simulink library "MIL_Test"  (Simulink 7.0)
values from neighbouring files (symbols this model uses):
  TID = min('TI' == AFT(1:2))    [PAS_callback.m]    (also in PSTID_callback.m = [block '/TID'])
undefined symbols (not defined in the file or in its folder): getdatatypespecs, slcm, StepSize
libraries: simulink x71, MIL_Test x6
(part 2 of 11)

== system MIL_Test/Test Data/Feature generation/Generate  local maximum  with given slope ==
  Clock : Clock
      settings: DisableCoverage=on  Decimation=10
  Limited Ramp Increasing : Subsystem
  Limited Ramp  Decreasing1 : Subsystem
  Logical Operator : Logic  AllPortsSameDT=off  OutDataTypeMode=boolean
  NoStartOfSignal1 : Switch  Criteria=u2 > Threshold
  RO : RelationalOperator  Operator=<  LogicOutDataTypeMode=boolean
  Sum : Sum  Inputs=|++  OutDataType=sfix(16)  OutScaling=2^0
  XO : Constant  DisableCoverage=on  Value=X0  OutDataType=sfix(16)  OutScaling=2^0
  XO1 : Constant  DisableCoverage=on  Value=X0  OutDataType=sfix(16)  OutScaling=2^0
  startTimeOfMax : Constant  DisableCoverage=on  Value=maxt  OutDataType=sfix(16)  OutScaling=2^0
  stopped : RelationalOperator  Operator=>  LogicOutDataTypeMode=boolean
  Maximum : Outport  OutDataType=sfix(16)  OutScaling=2^0
  wires:
  Logical Operator/1 -> NoStartOfSignal1/2
  stopped/1 -> Logical Operator/2
  RO/1 -> Logical Operator/1
  XO1/1 -> RO/2
  startTimeOfMax/1 -> stopped/2
  Clock/1 -> stopped/1
  Limited Ramp Increasing/2(MaxValue2) -> Limited Ramp  Decreasing1/1(InitialValue)
  Limited Ramp Increasing/1(Out2) -> Sum/1
  NoStartOfSignal1/1 -> Maximum/1
  XO/1 -> NoStartOfSignal1/1
  Sum/1 -> NoStartOfSignal1/3
  Limited Ramp  Decreasing1/1(Out1) -> RO/1, Sum/2

== system MIL_Test/Test Data/Feature generation/Generate  local maximum = maxvalue  @ given time ==
  Repeating Sequence : simulink/Sources/Repeating Sequence  SystemSampleTime=-1  rep_seq_t=[0 maxt maxt+1]  rep_seq_y=[X0 maxv X0]
  Maximum : Outport  OutDataType=sfix(16)  OutScaling=2^0
  wires:
  Repeating Sequence/1 -> Maximum/1

== system MIL_Test/Test Data/Feature generation/Generate any step response  characteristics ==
  Plant : TransferFcn  Numerator=[10]  Denominator=[1 1 10]
  Scope : Scope  NumInputPorts=5
      settings: YMin=-5~-5~-5~-5~-5  YMax=5~5~5~5~5  MaxDataPoints=1115000
  Step1 : Step  Time=2  SampleTime=0
  Sum : Sum  Inputs=|+-  OutDataType=sfix(16)  OutScaling=2^0
  Step response : Outport  OutDataType=sfix(16)  OutScaling=2^0
  wires:
  Sum/1 -> Plant/1
  Step1/1 -> Sum/1  "Step"
  Plant/1 -> Step response/1, Sum/2, Scope/1  "Step response"

== system MIL_Test/Test Data/Feature generation/Generate complete step ==
  InOut Bus : Inport  OutDataType=sfix(16)  OutScaling=2^0
  Bus Selector : BusSelector  OutputSignals=signal2.T
  Clock1 : Clock
      settings: Decimation=10
  Data Store : DataStoreMemory  StartFcn=triggerTime=triggerTime +50;  DataStoreName=triggerTime  OutDataType=sfix(16)  OutScaling=2^0
  Generate step : Step  InitFcn=triggerTime=0;  StartFcn=triggerTime=triggerTime+50;  Time=150  Before=100  After=40  SampleTime=0
  Generate step1 : Step  Time=100  Before=80  After=100  SampleTime=0
  Hold Time : Subsystem  TreatAsAtomicUnit=on
  Hold Value : Subsystem  TreatAsAtomicUnit=on
  Memory : Memory
  Relational Operator : RelationalOperator  Operator===  LogicOutDataTypeMode=boolean
  Switch : Switch  Criteria=u2 > Threshold
  triggered : Constant  OutDataType=sfix(16)  OutScaling=2^0
  v_Des : Outport  OutDataType=sfix(16)  OutScaling=2^0
  wires:
  Bus Selector/1 -> Memory/1  "<T>"
  Memory/1 -> Relational Operator/1
  Clock1/1 -> Hold Time/1(Clock)
  Hold Value/1(v_Des) -> Switch/2
  Switch/1 -> v_Des/1
  Generate step1/1 -> Switch/3
  Generate step/1 -> Switch/1
  Relational Operator/1 -> Hold Time/Enable, Hold Value/Enable, Hold Value/1(In1)
  triggered/1 -> Relational Operator/2
  InOut Bus/1 -> Bus Selector/1

== system MIL_Test/Test Data/Feature generation/Generate linear relation ==
  Clock : Clock
      settings: DisableCoverage=on  Decimation=10
  Product : Product  DisableCoverage=on  OutDataType=sfix(16)  OutScaling=2^0  SaturateOnIntegerOverflow=on  InputSameDT=on
  Step : Step  DisableCoverage=on  Time=0  After=c  SampleTime=0
  Out1 : Outport  OutDataType=sfix(16)  OutScaling=2^0
  wires:
  Clock/1 -> Product/2
  Product/1 -> Out1/1
  Step/1 -> Product/1

== system MIL_Test/Test Data/Feature generation/Generate min to date ==
  Sine Wave : Sin  SampleTime=0
  Step1 : Step  Time=2  SampleTime=0
  Step2 : Step  Time=5  Before=up  After=low  SampleTime=0
  Sum : Sum  Inputs=|+++  OutDataType=sfix(16)  OutScaling=2^0
  Min to date : Outport  OutDataType=sfix(16)  OutScaling=2^0
  wires:
  Step1/1 -> Sum/1  "Step"
  Sum/1 -> Min to date/1
  Step2/1 -> Sum/2
  Sine Wave/1 -> Sum/3

== system MIL_Test/Test Data/Feature generation/Generate peaks ==
  Repeating Sequence : simulink/Sources/Repeating Sequence  SystemSampleTime=-1  rep_seq_t=[0 1/freq]  rep_seq_y=[Sens -Sens]
  Peak : Outport  OutDataType=sfix(16)  OutScaling=2^0
  wires:
  Repeating Sequence/1 -> Peak/1

== system MIL_Test/Test Data/Feature generation/Generate signal  crossing a given value  @ given time ==
  Step : Step  Time=time  Before=up-low+1  After=val  SampleTime=0
  Feature : Outport  OutDataType=sfix(16)  OutScaling=2^0
  wires:
  Step/1 -> Feature/1

== system MIL_Test/Test Data/Feature generation/Generate signal which  starts to be constant @ time ==
  Clock1 : Clock
      settings: Decimation=10
  Constant : Constant  Value=const  OutDataType=sfix(16)  OutScaling=2^0
  Relational Operator : RelationalOperator  LogicOutDataTypeMode=boolean
  Sine Wave : Sin  SampleTime=0
  Switch1 : Switch  Criteria=u2 > Threshold
  start time : Constant  Value=ST  OutDataType=sfix(16)  OutScaling=2^0
  Feature : Outport  OutDataType=sfix(16)  OutScaling=2^0
  wires:
  Clock1/1 -> Relational Operator/1
  start time/1 -> Relational Operator/2
  Relational Operator/1 -> Switch1/2
  Constant/1 -> Switch1/1
  Sine Wave/1 -> Switch1/3
  Switch1/1 -> Feature/1

== system MIL_Test/Test Data/Feature generation/Generate timed constant ==
  Repeating Sequence : Subsystem  mask(Repeating table){rep_seq_t=[0 T], rep_seq_y=[X0 X0]}
      mask prompts: rep_seq_t "Time values:"; rep_seq_y "Output values:"
      mask help: Output a repeating sequence of numbers specified in a table of time-value pairs. Values of time should be monotonically increasing.
      mask init:
      | if (length(rep_seq_t) ~= length(rep_seq_y)),
      |   error('Length of time vector and output vector must be the same.')
      | end
      | dbl_rep_seq_t = double(rep_seq_t);
      | dbl_rep_seq_y = double(rep_seq_y);
      | period = max(dbl_rep_seq_t) - min(dbl_rep_seq_t);
      | s = round(length(dbl_rep_seq_t)/50);
      | if s > 0
      |   pts = [1:s:length(dbl_rep_seq_t)];
      |   L   = length(pts);
      | else
      |   L   = length(dbl_rep_seq_t);
      |   pts = [1:L];
      | end
      | 
      | disp_seq_t = reshape(dbl_rep_seq_t(pts),L,1);
      | disp_seq_y = reshape(dbl_rep_seq_y(pts),L,1);
      | disp_period = max(disp_seq_t) - min(disp_seq_t);
      | 
      | disp_seq_t  = repmat(disp_seq_t,1,3) + (ones(L,1)*(disp_period*[0,1,2]));
      | disp_seq_t = [ disp_seq_t(:); disp_seq_t(end) ];
      | disp_seq_y = repmat(disp_seq_y,1,3);
      | disp_seq_y = [ disp_seq_y(:); disp_seq_y(1) ];
      mask Help: Repeats cycle given in table. Time values should be monotonically increasing.
      mask Display: plot( disp_seq_t, disp_seq_y )
  Out1 : Outport  OutDataType=sfix(16)  OutScaling=2^0
  wires:
  Repeating Sequence/1(Out1) -> Out1/1

== system MIL_Test/Test Data/Feature generation/Generate timed limited decrease ==
  Clock : Clock
      settings: Decimation=10
  Constant : Constant  Value=start  OutDataType=sfix(16)  OutScaling=2^0
  Constant1 : Constant  Value=X0  OutDataType=sfix(16)  OutScaling=2^0
  Constant2 : Constant  Value=XF  OutDataType=sfix(16)  OutScaling=2^0
  Output : Sum  Inputs=|++  OutDataType=sfix(16)  OutScaling=2^0  SaturateOnIntegerOverflow=on  InputSameDT=on
  Product : Product  OutDataType=sfix(16)  OutScaling=2^0  SaturateOnIntegerOverflow=on  InputSameDT=on
  Step : Step  Time=start  After=(XF-X0)/T  SampleTime=0
  Subsystem : Subsystem
  Sum : Sum  Inputs=|+-  OutDataType=sfix(16)  OutScaling=2^0  SaturateOnIntegerOverflow=on  InputSameDT=on
  Out1 : Outport  OutDataType=sfix(16)  OutScaling=2^0
  wires:
  Constant2/1 -> Subsystem/1(In1)
  Step/1 -> Product/1
  Product/1 -> Output/1
  Constant1/1 -> Output/2, Subsystem/3(In3)
  Output/1 -> Subsystem/2(In2)
  Sum/1 -> Product/2
  Constant/1 -> Sum/2
  Clock/1 -> Sum/1
  Subsystem/1(Out1) -> Out1/1

== system MIL_Test/Test Data/Feature generation/Generate timed limited increase ==
  Clock : Clock
      settings: Decimation=10
  Constant : Constant  Value=start  OutDataType=sfix(16)  OutScaling=2^0
  Constant1 : Constant  Value=X0  OutDataType=sfix(16)  OutScaling=2^0
  Constant2 : Constant  Value=XF  OutDataType=sfix(16)  OutScaling=2^0
  Output : Sum  Inputs=|++  OutDataType=sfix(16)  OutScaling=2^0  SaturateOnIntegerOverflow=on  InputSameDT=on
  Product : Product  OutDataType=sfix(16)  OutScaling=2^0  SaturateOnIntegerOverflow=on  InputSameDT=on
  Step : Step  Time=start  After=(XF-X0)/T  SampleTime=0
  Subsystem : Subsystem
  Sum : Sum  Inputs=|+-  OutDataType=sfix(16)  OutScaling=2^0  SaturateOnIntegerOverflow=on  InputSameDT=on
  Out1 : Outport  OutDataType=sfix(16)  OutScaling=2^0
  wires:
  Step/1 -> Product/1
  Product/1 -> Output/1
  Constant1/1 -> Output/2, Subsystem/3(In3)
  Sum/1 -> Product/2
  Constant/1 -> Sum/2
  Clock/1 -> Sum/1
  Constant2/1 -> Subsystem/1(In1)
  Output/1 -> Subsystem/2(In2)  "U(k)"
  Subsystem/1(Out1) -> Out1/1

== system MIL_Test/Test Data/Signal comparison/Bound Precond ==
  Signal : Inport  OutDataType=sfix(16)  OutScaling=2^0
  Reference : Inport  Port=2  OutDataType=sfix(16)  OutScaling=2^0
  RelOp : RelationalOperator  LogicOutDataTypeMode=Specify via dialog
  Activate : Outport  OutDataType=sfix(16)  OutScaling=2^0
  wires:
  Reference/1 -> RelOp/2
  RelOp/1 -> Activate/1
  Signal/1 -> RelOp/1

== system MIL_Test/Test Data/Signal comparison/Range - Gap Absolute tolerance Precond ==
  Signal : Inport  OutDataType=sfix(16)  OutScaling=2^0
  Reference : Inport  Port=2  OutDataType=sfix(16)  OutScaling=2^0
  Abs : Abs
  Abs1 : Abs
  Absolute Tolerance : Constant  Value=AbsoluteTolerance  OutDataType=sfix(16)  OutScaling=2^0
  Add : Sum  Inputs=+-  OutDataType=sfix(16)  OutScaling=2^-10
  Relational Operator : RelationalOperator  Operator===  LogicOutDataTypeMode=boolean
  Activate : Outport  OutDataType=sfix(16)  OutScaling=2^0
  wires:
  Abs1/1 -> Relational Operator/2
  Absolute Tolerance/1 -> Abs1/1
  Reference/1 -> Add/2
  Signal/1 -> Add/1
  Add/1 -> Abs/1
  Abs/1 -> Relational Operator/1
  Relational Operator/1 -> Activate/1

== system MIL_Test/Test Data/Signal comparison/Range - Gap Relative tolerance Precond ==
  Signal : Inport  OutDataType=sfix(16)  OutScaling=2^0
  Reference : Inport  Port=2  OutDataType=sfix(16)  OutScaling=2^0
  Abs : Abs
  Abs1 : Abs
  Add : Sum  Inputs=+-  OutDataType=sfix(16)  OutScaling=2^-10
  Divide1 : Product  Inputs=**/  OutDataType=sfix(16)  OutScaling=2^-10
  Max : Constant  Value=100  OutDataType=sfix(16)  OutScaling=2^0
  Relational Operator : RelationalOperator  Operator=<=  LogicOutDataTypeMode=boolean
  Relative Tolerance : Constant  OutDataType=sfix(16)  OutScaling=2^0
  Activate : Outport  OutDataType=sfix(16)  OutScaling=2^0
  wires:
  Abs/1 -> Relational Operator/1
  Add/1 -> Abs/1
  Signal/1 -> Add/1
  Reference/1 -> Add/2, Abs1/1
  Divide1/1 -> Relational Operator/2
  Max/1 -> Divide1/3
  Relative Tolerance/1 -> Divide1/2
  Relational Operator/1 -> Activate/1
  Abs1/1 -> Divide1/1

== system MIL_Test/Test Data/Signal comparison/Range - Gap Tolerance range Precond ==
  Signal : Inport  OutDataType=sfix(16)  OutScaling=2^0
  Lower bound : Inport  Port=2  OutDataType=sfix(16)  OutScaling=2^0
  Upper bound : Inport  Port=3  OutDataType=sfix(16)  OutScaling=2^0
  Logical Operator : Logic  AllPortsSameDT=off  OutDataTypeMode=Specify via dialog
  Relational Operator : RelationalOperator  LogicOutDataTypeMode=boolean
  Relational Operator1 : RelationalOperator  LogicOutDataTypeMode=boolean
  Activate : Outport  OutDataType=sfix(16)  OutScaling=2^0
  wires:
  Upper bound/1 -> Relational Operator1/1
  Relational Operator/1 -> Logical Operator/2
  Relational Operator1/1 -> Logical Operator/1
  Signal/1 -> Relational Operator/1, Relational Operator1/2
  Logical Operator/1 -> Activate/1
  Lower bound/1 -> Relational Operator/2

== system MIL_Test/Test Data/Test Data Architecture/<Test data generator> ==
  Test Ctrl Influence : Inport  OutDataType=sfix(16)  OutScaling=2^0
  Out Bus : Inport  Port=2  OutDataType=sfix(16)  OutScaling=2^0
  <Requirement name> : Subsystem
  switch <signal1> : MultiPortSwitch  Inputs=1  zeroidx=on
  <signal1> : Outport  OutDataType=sfix(16)  OutScaling=2^0
  wires:
  Test Ctrl Influence/1 -> switch <signal1>/1
  Out Bus/1 -> <Requirement name>/1(Out Bus)
  switch <signal1>/1 -> <signal1>/1
  <Requirement name>/1(<signal1>) -> switch <signal1>/2

== system MIL_Test/Test Quality/VFs Activation  Coverage/Max to date ==
  Signal : Inport  OutDataType=sfix(16)  OutScaling=2^0
  Clock : Clock
      settings: Decimation=10
  Memory : Memory  Orientation=left
  MinMax : MinMax  Function=max  Inputs=2  OutDataType=sfix(16)  OutScaling=2^0
  Switch : Switch  Criteria=u2 > Threshold
  Max : Outport  OutDataType=sfix(16)  OutScaling=2^0
  wires:
  Memory/1 -> Switch/1
  Clock/1 -> Switch/2
  Switch/1 -> MinMax/1
  Signal/1 -> Switch/3, MinMax/2
  MinMax/1 -> Memory/1, Max/1

== system MIL_Test/Test Quality/VFs Activation  Coverage/Max to date1 ==
  Signal : Inport  OutDataType=sfix(16)  OutScaling=2^0
  Clock : Clock
      settings: Decimation=10
  Memory : Memory  Orientation=left
  MinMax : MinMax  Function=max  Inputs=2  OutDataType=sfix(16)  OutScaling=2^0
  Switch : Switch  Criteria=u2 > Threshold
  Max : Outport  OutDataType=sfix(16)  OutScaling=2^0
  wires:
  Memory/1 -> Switch/1
  Clock/1 -> Switch/2
  Switch/1 -> MinMax/1
  Signal/1 -> Switch/3, MinMax/2
  MinMax/1 -> Memory/1, Max/1

== system MIL_Test/Validation Function/Feature extraction/Complete step detection ==
  Step : Inport  OutDataType=sfix(16)  OutScaling=2^0
  Step response : Inport  Port=2  OutDataType=sfix(16)  OutScaling=2^0
  Step detection : Subsystem  mask{MT=10, RT=0.001}
      mask prompts: MT "Minimal time for signals to be constant before a step"; RT "Relative tolerance for constant detection in %"
      mask CallbackString:
      | if (str2double(get_param(gcb,'MT')) < 0)
      |     error(['Minimal time specified (' get_param(gcb,'MT') ') negative. Please give a non-negative value.']);
      | else
      |     set_param([gcb '/Active if signals constant for some specified time/Min Time'],'Value',get_param(gcb,'MT'));
      | end|if or( (str2double(get_param(gcb,'RT')) < 0), (str2double(get_param(gcb,'RT')) > 100))
      |     error(['Relative tolerance value (' get_param(gcb,'RT') ') out of range. Please give a value between 0 and 100.']);
      | else
      |     set_param([gcb '/Active if signals constant for some specified time/Time since signal constant/Detect constant/Relative tolerance/Relative Tolerance'],'Value',get_param(gcb,'RT'));
      |     set_param([gcb '/Active if signals constant for some specified time/Time since signal constant/Detect constant'],'RT',get_param(gcb,'RT'));
      |     set_param([gcb '/Active if signals constant for some specified time/Time since signal constant'],'RT',get_param(gcb,'RT'));
      |     set_param([gcb '/Active if signals constant for some specified time/Time since signal constant1/Detect constant/Relative tolerance/Relative Tolerance'],'Value',get_param(gcb,'RT'));
      |     set_param([gcb '/Active if signals constant for some specified time/Time since signal constant1/Detect constant'],'RT',get_param(gcb,'RT'));
      |     set_param([gcb '/Active if signals constant for some specified time/Time since signal constant1'],'RT',get_param(gcb,'RT'));
      | end
  Step detection reset : Subsystem  mask{MT=10, RT=0.0001, MSS=10}
      mask prompts: MT "Minimal time for signals to be constant before a step"; RT "Relative tolerance for constant detection in %"; MSS "Minimal step size for step detection"
      mask CallbackString:
      | if (str2double(get_param(gcb,'MT')) < 0)
      |     error(['Minimal time specified (' get_param(gcb,'MT') ') negative. Please give a non-negative value.']);
      | else
      |     set_param([gcb '/Active if signals constant for some specified time/Min Time'],'Value',get_param(gcb,'MT'));
      | end|if or( (str2double(get_param(gcb,'RT')) < 0), (str2double(get_param(gcb,'RT')) > 100))
      |     error(['Relative tolerance value (' get_param(gcb,'RT') ') out of range. Please give a value between 0 and 100.']);
      | else
      |     set_param([gcb '/Active if signals constant for some specified time/Time since signal constant/Detect constant/Relative tolerance/Relative Tolerance'],'Value',get_param(gcb,'RT'));
      |     set_param([gcb '/Active if signals constant for some specified time/Time since signal constant/Detect constant'],'RT',get_param(gcb,'RT'));
      |     set_param([gcb '/Active if signals constant for some specified time/Time since signal constant'],'RT',get_param(gcb,'RT'));
      |     set_param([gcb '/Active if signals constant for some specified time/Time since signal constant1/Detect constant/Relative tolerance/Relative Tolerance'],'Value',get_param(gcb,'RT'));
      |     set_param([gcb '/Active if signals constant for some specified time/Time since signal constant1/Detect constant'],'RT',get_param(gcb,'RT'));
      |     set_param([gcb '/Active if signals constant for some specified time/Time since signal constant1'],'RT',get_param(gcb,'RT'));
      | end|if (str2double(get_param(gcb,'MSS')) < 0)
      |     error(['Minimal step size specified (' get_param(gcb,'MSS') ') negative. Please give a non-negative value.']);
      | else
      |     set_param([gcb '/Step detection/Min step size'],'Value',get_param(gcb,'MSS'));
      |     set_param([gcb '/Step detection'],'StepSize',get_param(gcb,'MSS'));
      | 
      | end
  R : Outport  OutDataType=sfix(16)  OutScaling=2^0
  T : Outport  Port=2  OutDataType=sfix(16)  OutScaling=2^0
  Complete step : Outport  Port=3  OutDataType=sfix(16)  OutScaling=2^0
  wires:
  Step detection/1(End of complete step) -> T/1, Complete step/1
  Step detection reset/1(R) -> R/1, Step detection/1(R)
  Step response/1 -> Step detection reset/2(Step response), Step detection/3(Step response)
  Step/1 -> Step detection reset/1(Step), Step detection/2(Step)

== system MIL_Test/Validation Function/Feature extraction/Detect constant ==
  Signal : Inport  OutDataType=sfix(16)  OutScaling=2^0
  Clock : Clock
      settings: Decimation=10
  Constant1 : Constant  Value=0  OutDataTypeMode=boolean  OutDataType=sfix(16)  OutScaling=2^0
  Memory : Memory
  Relative tolerance : Subsystem
  Switch : Switch  Criteria=u2 > Threshold
  Constant : Outport  OutDataType=sfix(16)  OutScaling=2^0
  wires:
  Switch/1 -> Constant/1
  Relative tolerance/1(sig == ref) -> Switch/1
  Clock/1 -> Switch/2
  Constant1/1 -> Switch/3
  Memory/1 -> Relative tolerance/2(ref)
  Signal/1 -> Relative tolerance/1(sig), Memory/1

== system MIL_Test/Validation Function/Feature extraction/Detect decrease ==
  Signal : Inport  OutDataType=sfix(16)  OutScaling=2^0
  Clock : Clock
      settings: Decimation=10
  Memory : Memory
  Relational Operator : RelationalOperator  Operator=<  LogicOutDataTypeMode=Specify via dialog
  Switch : Switch  Criteria=u2 > Threshold
  Decrease : Outport  OutDataType=sfix(16)  OutScaling=2^0
  wires:
  Signal/1 -> Relational Operator/1, Memory/1, Switch/3
  Relational Operator/1 -> Decrease/1
  Clock/1 -> Switch/2
  Memory/1 -> Switch/1
  Switch/1 -> Relational Operator/2

== system MIL_Test/Validation Function/Feature extraction/Detect increase ==
  Signal : Inport  OutDataType=sfix(16)  OutScaling=2^0
  Clock : Clock
      settings: Decimation=10
  Memory : Memory
  Relational Operator : RelationalOperator  Operator=>  LogicOutDataTypeMode=Specify via dialog
  Switch : Switch  Criteria=u2 > Threshold
  Increase : Outport  OutDataType=sfix(16)  OutScaling=2^0
  wires:
  Switch/1 -> Relational Operator/2
  Memory/1 -> Switch/1
  Clock/1 -> Switch/2
  Relational Operator/1 -> Increase/1
  Signal/1 -> Switch/3, Memory/1, Relational Operator/1

== system MIL_Test/Validation Function/Feature extraction/Linear relation ==
  y : Inport  OutDataType=sfix(16)  OutScaling=2^0
  u : Inport  Port=2  OutDataType=sfix(16)  OutScaling=2^0
  Product : Product  OutDataType=sfix(16)  OutScaling=2^0  RndMeth=Zero
  Relative tolerance : Subsystem
  c : Constant  Value=5  OutDataType=sfix(16)  OutScaling=2^0
  y == c u : Outport  OutDataType=sfix(16)  OutScaling=2^0
  wires:
  Relative tolerance/1(sig == ref) -> y == c u/1
  c/1 -> Product/2
  u/1 -> Product/1
  Product/1 -> Relative tolerance/2(ref)
  y/1 -> Relative tolerance/1(sig)

== system MIL_Test/Validation Function/Feature extraction/Local maximum ==
  Signal : Inport  OutDataType=sfix(16)  OutScaling=2^0
  Clock : Clock
      settings: Decimation=10
  Clock1 : Clock
      settings: Decimation=10
  Logical Operator : Logic  AllPortsSameDT=off  OutDataTypeMode=boolean
  Memory : Memory
  Memory1 : Memory
  Relational Operator : RelationalOperator  Operator=<  LogicOutDataTypeMode=boolean
  Relational Operator1 : RelationalOperator  Operator=>  LogicOutDataTypeMode=boolean
  Switch : Switch  Criteria=u2 > Threshold
  Switch1 : Switch  Criteria=u2 > Threshold
  Maximum : Outport  OutDataType=sfix(16)  OutScaling=2^0
  wires:
  Switch1/1 -> Relational Operator1/2
  Memory1/1 -> Switch1/1
  Clock1/1 -> Switch1/2
  Switch/1 -> Relational Operator1/1, Switch1/3, Memory1/1, Relational Operator/2
  Memory/1 -> Switch/1
  Clock/1 -> Switch/2
  Relational Operator/1 -> Logical Operator/1
  Relational Operator1/1 -> Logical Operator/2
  Logical Operator/1 -> Maximum/1
  Signal/1 -> Switch/3, Memory/1, Relational Operator/1

== system MIL_Test/Validation Function/Feature extraction/Min to date ==
  Signal : Inport  OutDataType=sfix(16)  OutScaling=2^0
  Clock : Clock
      settings: Decimation=10
  Memory : Memory  Orientation=left
  MinMax : MinMax  Inputs=2  OutDataType=sfix(16)  OutScaling=2^0
  Switch : Switch  Criteria=u2 > Threshold
  Min : Outport  OutDataType=sfix(16)  OutScaling=2^0
  wires:
  Memory/1 -> Switch/1
  Clock/1 -> Switch/2
  Switch/1 -> MinMax/1
  Signal/1 -> Switch/3, MinMax/2
  MinMax/1 -> Memory/1, Min/1

== system MIL_Test/Validation Function/Feature extraction/Moving average ==
  Signal : Inport  OutDataType=sfix(16)  OutScaling=2^0
  Add : Sum  OutDataType=sfix(16)  OutScaling=2^-10
  Clock : Clock
      settings: Decimation=10
  Constant : Constant  Value=2  OutDataType=sfix(16)  OutScaling=2^0
  Divide : Product  Inputs=*/  OutDataType=sfix(16)  OutScaling=2^-10
  Memory : Memory
  Switch : Switch  Criteria=u2 > Threshold
  MA : Outport  OutDataType=sfix(16)  OutScaling=2^0
  wires:
  Switch/1 -> Add/2
  Memory/1 -> Switch/1
  Clock/1 -> Switch/2
  Signal/1 -> Add/1, Switch/3, Memory/1
  Add/1 -> Divide/1
  Constant/1 -> Divide/2
  Divide/1 -> MA/1

== system MIL_Test/Validation Function/Feature extraction/Peak detection ==
  Signal : Inport  OutDataType=sfix(16)  OutScaling=2^0
  Abs : Abs
  Abs1 : Abs
  Add : Sum  Inputs=+-  OutDataType=sfix(16)  OutScaling=2^-10
  Add1 : Sum  Inputs=+-  OutDataType=sfix(16)  OutScaling=2^-10
  Clock : Clock
      settings: Decimation=10
  Clock1 : Clock
      settings: Decimation=10
  Compare To Zero : simulink/Logic and Bit Operations/Compare To Zero  SystemSampleTime=-1  relop=<=  LogicOutDataTypeMode=boolean  ZeroCross=off
  Logical Operator : Logic  Inputs=3  AllPortsSameDT=off  OutDataTypeMode=boolean
  Memory : Memory
  Memory1 : Memory
  Product : Product  OutDataType=sfix(16)  OutScaling=2^0  RndMeth=Zero
  Relational Operator : RelationalOperator  Operator=<=  LogicOutDataTypeMode=boolean
  Relational Operator1 : RelationalOperator  LogicOutDataTypeMode=boolean
  Sensibility1 : Constant  Value=0.198  OutDataType=sfix(16)  OutScaling=2^0
  Sensibility2 : Constant  Value=0.198  OutDataType=sfix(16)  OutScaling=2^0
  Switch : Switch  Criteria=u2 > Threshold
  Switch1 : Switch  Criteria=u2 > Threshold
  Peak : Outport  OutDataType=sfix(16)  OutScaling=2^0
  wires:
  Sensibility2/1 -> Relational Operator1/2
  Abs1/1 -> Relational Operator1/1
  Sensibility1/1 -> Relational Operator/1
  Abs/1 -> Relational Operator/2
  Product/1 -> Compare To Zero/1
  Compare To Zero/1 -> Logical Operator/2
  Relational Operator1/1 -> Logical Operator/3
  Relational Operator/1 -> Logical Operator/1
  Add1/1 -> Product/2, Abs1/1
  Signal/1 -> Memory/1, Switch/3, Add/1
  Logical Operator/1 -> Peak/1
  Clock/1 -> Switch/2
  Memory/1 -> Switch/1
  Switch/1 -> Add1/1, Add/2, Memory1/1, Switch1/3
  Clock1/1 -> Switch1/2
  Memory1/1 -> Switch1/1
  Switch1/1 -> Add1/2
  Add/1 -> Product/1, Abs/1

== system MIL_Test/Validation Function/Feature extraction/Signal value @ maximum ==
  Signal : Inport  OutDataType=sfix(16)  OutScaling=2^0
  Local maximum : Subsystem  TreatAsAtomicUnit=on
  Trigger : Outport  OutDataType=sfix(16)  OutScaling=2^0
  Feature : Outport  Port=2  OutDataType=sfix(16)  OutScaling=2^0
  wires:
  Local maximum/1(Maximum) -> Trigger/1
  Signal/1 -> Local maximum/1(Signal), Feature/1

== system MIL_Test/Validation Function/Feature extraction/Step detection ==
  Signal : Inport  OutDataType=sfix(16)  OutScaling=2^0
  Abs : Abs
  Add : Sum  Inputs=+-  OutDataType=sfix(16)  OutScaling=2^-10
  Clock : Clock
      settings: Decimation=10
  Memory : Memory
  Min step size : Constant  OutDataType=sfix(16)  OutScaling=2^0
  Relational Operator : RelationalOperator  LogicOutDataTypeMode=boolean
  Switch : Switch  Criteria=u2 > Threshold
  Step : Outport  OutDataType=sfix(16)  OutScaling=2^0
  wires:
  Switch/1 -> Add/2
  Memory/1 -> Switch/1
  Clock/1 -> Switch/2
  Signal/1 -> Add/1, Switch/3, Memory/1
  Abs/1 -> Relational Operator/1
  Min step size/1 -> Relational Operator/2
  Relational Operator/1 -> Step/1
  Add/1 -> Abs/1

== system MIL_Test/Validation Function/Feature extraction/Step response characteristics ==
  Step : Inport  OutDataType=sfix(16)  OutScaling=2^0
  Step response : Inport  Port=2  OutDataType=sfix(16)  OutScaling=2^0
  Step response characteristics extraction : Subsystem  mask(Step response feature extraction){gain=0.8333, lowerLim=10, upperLim=90, MOma=ones(1,10), RelTol=0.1, MinTime=1, Range=5, sseW=ones(1,10)}
      mask prompts: gain "System's static gain"; lowerLim "Rise time interval lower limit (in set point %)"; upperLim "Rise time interval upper limit (in set point %)"; MOma "Maximum overshoot moving average weights"; RelTol "Maximum overshoot - Detect constant if no overshoot - Relative Tolerance"; MinTime "Maximum overshoot - Detect constant if no overshoot - Minimum constant time"; Range "Settling time range (in set point %)"; sseW "Steady state error - moving average weights"
      mask help: Extracts four step response feature characteristics. Extraction parameters are shown below.
      mask CallbackString:
      | set_param([gcb '/Static Gain'],'Value',get_param(gcb,'gain'));|set_param([gcb '/Extract rise time/lowerLim'],'Value',get_param(gcb,'lowerLim'));|set_param([gcb '/Extract rise time/upperLim'],'Value',get_param(gcb,'upperLim'));|set_param([gcb '/Extract maximum overshoot/Step response moving average and initial conditions before step/Weighted Moving Average'],'mgainval',get_param(gcb,'MOma'));
      | set_param([gcb '/Extract maximum overshoot/Step response moving average and initial conditions before step/Weighted Moving Average1'],'mgainval',get_param(gcb,'MOma'));|set_param([gcb '/Extract maximum overshoot/Active if signals constant for some specified time/Time since signal constant'],'RT',get_param(gcb,'RelTol'));
      | set_param([gcb '/Extract maximum overshoot/Active if signals constant for some specified time/Time since signal constant1'],'RT',get_param(gcb,'RelTol'));|set_param([gcb '/Extract maximum overshoot/Active if signals constant for some specified time/Min Time'],'Value',get_param(gcb,'MinTime'));|set_param([gcb '/Extract settling time/Set point percent'],'Value',get_param(gcb,'Range'));|set_param([gcb '/Extract steady state error/Weighted Moving Average'],'mgainval',get_param(gcb,'sseW'));
  Step response reset : Subsystem  mask{MT=1, RT=0.0001, MSS=1}
      mask prompts: MT "Minimal time for signals to be constant before a step"; RT "Relative tolerance for constant detection in %"; MSS "Minimal step size for step detection"
      mask CallbackString:
      | if (str2double(get_param(gcb,'MT')) < 0)
      |     error(['Minimal time specified (' get_param(gcb,'MT') ') negative. Please give a non-negative value.']);
      | else
      |     set_param([gcb '/Active if signals constant for some specified time/Min Time'],'Value',get_param(gcb,'MT'));
      | end|if or( (str2double(get_param(gcb,'RT')) < 0), (str2double(get_param(gcb,'RT')) > 100))
      |     error(['Relative tolerance value (' get_param(gcb,'RT') ') out of range. Please give a value between 0 and 100.']);
      | else
      |     set_param([gcb '/Active if signals constant for some specified time/Time since signal constant/Detect constant/Relative tolerance/Relative Tolerance'],'Value',get_param(gcb,'RT'));
      |     set_param([gcb '/Active if signals constant for some specified time/Time since signal constant/Detect constant'],'RT',get_param(gcb,'RT'));
      |     set_param([gcb '/Active if signals constant for some specified time/Time since signal constant'],'RT',get_param(gcb,'RT'));
      |     set_param([gcb '/Active if signals constant for some specified time/Time since signal constant1/Detect constant/Relative tolerance/Relative Tolerance'],'Value',get_param(gcb,'RT'));
      |     set_param([gcb '/Active if signals constant for some specified time/Time since signal constant1/Detect constant'],'RT',get_param(gcb,'RT'));
      |     set_param([gcb '/Active if signals constant for some specified time/Time since signal constant1'],'RT',get_param(gcb,'RT'));
      | end|if (str2double(get_param(gcb,'MSS')) < 0)
      |     error(['Minimal step size specified (' get_param(gcb,'MSS') ') negative. Please give a non-negative value.']);
      | else
      |     set_param([gcb '/Step detection/Min step size'],'Value',get_param(gcb,'MSS'));
      |     set_param([gcb '/Step detection'],'StepSize',get_param(gcb,'MSS'));
      | 
      | end
  Step response trigger : Subsystem  mask(Step response trigger extraction){MinTime=1, RelTol=0.5, MAXsse=0.5}
      mask prompts: MinTime "Detect constant signals - Minimum constant time"; RelTol "Detect constant signals - Relative Tolerance"; MAXsse "Maximum steady state error for triggering"
      mask help: This block extracts the trigger signals for the four step response characteristics.
      mask CallbackString:
      | set_param([gcb '/Active if signals constant for some specified time/Min Time'],'Value',get_param(gcb,'MinTime'));|set_param([gcb '/Active if signals constant for some specified time/Time since signal constant'],'RT',get_param(gcb,'RelTol'));
      | set_param([gcb '/Active if signals constant for some specified time/Time since signal constant1'],'RT',get_param(gcb,'RelTol'));|set_param([gcb '/Compare To Constant'],'const',get_param(gcb,'MAXsse'));
  R : Outport  OutDataType=sfix(16)  OutScaling=2^0
  Rise time T : Outport  Port=2  DataType=double  OutDataType=sfix(16)  OutScaling=2^0
  Overshoot T : Outport  Port=3  DataType=double  OutDataType=sfix(16)  OutScaling=2^0
  Settling time T : Outport  Port=4  DataType=double  OutDataType=sfix(16)  OutScaling=2^0
  Steady state error T : Outport  Port=5  DataType=double  OutDataType=sfix(16)  OutScaling=2^0
  Rise time : Outport  Port=6  OutDataType=sfix(16)  OutScaling=2^0
  Maximum Overshoot : Outport  Port=7  OutDataType=sfix(16)  OutScaling=2^0
  Settling time : Outport  Port=8  DataType=double  OutDataType=sfix(16)  OutScaling=2^0
  Steady state error : Outport  Port=9  DataType=double  OutDataType=sfix(16)  OutScaling=2^0
  wires:
  Step response trigger/4(Steady state error T) -> Steady state error T/1
  Step response trigger/3(Settling time T) -> Settling time T/1
  Step response trigger/2(Overshoot T) -> Overshoot T/1
  Step response trigger/1(Rise time T) -> Rise time T/1
  Step response characteristics extraction/2(Maximum overshoot) -> Maximum Overshoot/1
  Step response characteristics extraction/3(Settling time) -> Settling time/1
  Step response characteristics extraction/1(Rise time) -> Rise time/1
  Step response/1 -> Step response trigger/2(Step response), Step response characteristics extraction/3(Step response), Step response reset/2(Step response)
  Step/1 -> Step response characteristics extraction/2(Step), Step response reset/1(Step)
  Step response characteristics extraction/4(Steady state error) -> Steady state error/1, Step response trigger/1(Steady state error)
  Step response reset/1(R) -> Step response characteristics extraction/1(R), R/1

== system MIL_Test/Validation Function/Feature extraction/Time @ sig = x ==
  Signal : Inport  OutDataType=sfix(16)  OutScaling=2^0
  Clock : Clock
      settings: Decimation=10
  Relative tolerance : Subsystem
  Trigger Value : Constant  Value=5  OutDataType=sfix(16)  OutScaling=2^0
  Trigger : Outport  OutDataType=sfix(16)  OutScaling=2^0
  Feature : Outport  Port=2  OutDataType=sfix(16)  OutScaling=2^0
  wires:
  Clock/1 -> Feature/1
  Trigger Value/1 -> Relative tolerance/2(ref)
  Signal/1 -> Relative tolerance/1(sig)
  Relative tolerance/1(sig == ref) -> Trigger/1

== system MIL_Test/Validation Function/Feature extraction/Time since signal constant ==
  Signal : Inport  OutDataType=sfix(16)  OutScaling=2^0
  Clock : Clock
      settings: Decimation=10
  Detect constant : Subsystem  TreatAsAtomicUnit=on  mask(Feature extraction block){RT=1}
      mask prompts: RT "Relative tolerance in %"
      mask help: Detect if the signal value is constant (using the last two signal values) allowing for a user-defined relative deviation
      mask CallbackString:
      | if or( (str2double(get_param(gcb,'RT')) < 0), (str2double(get_param(gcb,'RT')) > 100))
      |     error(['Relative tolerance value (' get_param(gcb,'RT') ') out of range. Please give a value between 0 and 100.']);
      | else
      |     set_param([gcb '/Relative tolerance/Relative Tolerance'],'Value',get_param(gcb,'RT'));
      | end
  Logical Operator : Logic  Operator=NAND  AllPortsSameDT=off  OutDataTypeMode=boolean
  Logical Operator1 : Logic  Operator=NOT  AllPortsSameDT=off  OutDataTypeMode=boolean
  Memory : Memory  Orientation=left
  Memory1 : Memory
  Subtract : Sum  Inputs=-+  OutDataType=sfix(16)  OutScaling=2^-10
  Switch : Switch  Criteria=u2 > Threshold
  Trigger : Outport  OutDataType=sfix(16)  OutScaling=2^0
  Feature : Outport  Port=2  OutDataType=sfix(16)  OutScaling=2^0
  wires:
  Logical Operator/1 -> Switch/2
  Logical Operator1/1 -> Logical Operator/2
  Memory1/1 -> Logical Operator1/1
  Memory/1 -> Switch/1
  Switch/1 -> Memory/1, Subtract/1
  Clock/1 -> Switch/3, Subtract/2
  Subtract/1 -> Feature/1
  Detect constant/1(Constant) -> Memory1/1, Logical Operator/1, Trigger/1
  Signal/1 -> Detect constant/1(Signal)

== system MIL_Test/Validation Function/Signal comparison/Bound Ass ==
  Signal : Inport  OutDataType=sfix(16)  OutScaling=2^0
  Reference : Inport  Port=2  OutDataType=sfix(16)  OutScaling=2^0
  Bus Creator : BusCreator  Inputs=5
  Data Type Conversion{,1..3} (4 alike) : DataTypeConversion  OutDataType=sfix(16)  OutScaling=2^0
  Delay : Constant  Value=0  OutDataType=sfix(16)  OutScaling=2^0
  LOWER : Constant  Value=Lower  OutDataTypeMode=int8  OutDataType=sfix(16)  OutScaling=2^0
  No Limit : Constant  Value=Inf  OutDataType=sfix(16)  OutScaling=2^0
  No limit : Constant  Value=-Inf  OutDataType=sfix(16)  OutScaling=2^0
  Relational Operator : RelationalOperator  Operator=<=  LogicOutDataTypeMode=boolean  LogicDataType=double
  Switch 2 : Switch  Criteria=u2 ~= 0
  Switch 3 : Switch  Criteria=u2 ~= 0
  UPPER : Constant  Value=Upper  OutDataTypeMode=int8  OutDataType=sfix(16)  OutScaling=2^0
  V : Outport  OutDataType=sfix(16)  OutScaling=2^0  InitialOutput=[2]
  wires:
  Relational Operator/1 -> Data Type Conversion/1
  Data Type Conversion3/1 -> Bus Creator/4  "Actual data"
  Data Type Conversion2/1 -> Bus Creator/3  "Expected upper limit"
  Data Type Conversion1/1 -> Bus Creator/2  "Expected lower limit"
  Data Type Conversion/1 -> Bus Creator/1  "Local verdict"
  Bus Creator/1 -> V/1
  Reference/1 -> Relational Operator/2, Switch 2/3, Switch 3/3
  Signal/1 -> Data Type Conversion3/1, Relational Operator/1
  UPPER/1 -> Switch 3/2
  No Limit/1 -> Switch 3/1
  LOWER/1 -> Switch 2/2
  No limit/1 -> Switch 2/1
  Switch 2/1 -> Data Type Conversion1/1
  Switch 3/1 -> Data Type Conversion2/1
  Delay/1 -> Bus Creator/5  "Delay"

== system MIL_Test/Validation Function/Signal comparison/Bound Precond ==
  Signal : Inport  OutDataType=sfix(16)  OutScaling=2^0
  Reference : Inport  Port=2  OutDataType=sfix(16)  OutScaling=2^0
  RelOp : RelationalOperator  LogicOutDataTypeMode=Specify via dialog
  Activate : Outport  OutDataType=sfix(16)  OutScaling=2^0
  wires:
  Signal/1 -> RelOp/1
  RelOp/1 -> Activate/1
  Reference/1 -> RelOp/2

== system MIL_Test/Validation Function/Signal comparison/Range - Gap Absolute tolerance Ass ==
  Signal : Inport  OutDataType=sfix(16)  OutScaling=2^0
  Reference : Inport  Port=2  OutDataType=sfix(16)  OutScaling=2^0
  Abs : Abs
  Abs1 : Abs
  Absolute Tolerance : Constant  Value=AbsoluteTolerance  OutDataType=sfix(16)  OutScaling=2^0
  Add : Sum  Inputs=+-  OutDataType=sfix(16)  OutScaling=2^-10
  Add1 : Sum  Inputs=+-  OutDataType=sfix(16)  OutScaling=2^-10
  Add2 : Sum  OutDataType=sfix(16)  OutScaling=2^-10
  Bus Creator : BusCreator  Inputs=5
  Data Type Conversion{,1..3} (4 alike) : DataTypeConversion  OutDataType=sfix(16)  OutScaling=2^0
  Delay : Constant  Value=0  OutDataType=sfix(16)  OutScaling=2^0
  Relational Operator : RelationalOperator  Operator===  LogicOutDataTypeMode=boolean
  V : Outport  OutDataType=sfix(16)  OutScaling=2^0  InitialOutput=[2]
  wires:
  Abs1/1 -> Relational Operator/2, Add2/2, Add1/2
  Absolute Tolerance/1 -> Abs1/1
  Reference/1 -> Add/2, Add2/1, Add1/1
  Signal/1 -> Add/1, Data Type Conversion3/1
  Add/1 -> Abs/1
  Abs/1 -> Relational Operator/1
  Relational Operator/1 -> Data Type Conversion/1
  Delay/1 -> Bus Creator/5  "Delay"
  Add2/1 -> Data Type Conversion2/1
  Add1/1 -> Data Type Conversion1/1
  Bus Creator/1 -> V/1
  Data Type Conversion/1 -> Bus Creator/1  "Local verdict"
  Data Type Conversion1/1 -> Bus Creator/2  "Expected lower limit"
  Data Type Conversion2/1 -> Bus Creator/3  "Expected upper limit"
  Data Type Conversion3/1 -> Bus Creator/4  "Actual data"

== system MIL_Test/Validation Function/Signal comparison/Range - Gap Absolute tolerance Precond ==
  Signal : Inport  OutDataType=sfix(16)  OutScaling=2^0
  Reference : Inport  Port=2  OutDataType=sfix(16)  OutScaling=2^0
  Abs : Abs
  Abs1 : Abs
  Absolute Tolerance : Constant  Value=AbsoluteTolerance  OutDataType=sfix(16)  OutScaling=2^0
  Add : Sum  Inputs=+-  OutDataType=sfix(16)  OutScaling=2^-10
  Relational Operator : RelationalOperator  Operator===  LogicOutDataTypeMode=boolean
  Activate : Outport  OutDataType=sfix(16)  OutScaling=2^0
  wires:
  Relational Operator/1 -> Activate/1
  Abs/1 -> Relational Operator/1
  Add/1 -> Abs/1
  Signal/1 -> Add/1
  Reference/1 -> Add/2
  Absolute Tolerance/1 -> Abs1/1
  Abs1/1 -> Relational Operator/2

== system MIL_Test/Validation Function/Signal comparison/Range - Gap Relative tolerance Ass ==
  Signal : Inport  OutDataType=sfix(16)  OutScaling=2^0
  Reference : Inport  Port=2  OutDataType=sfix(16)  OutScaling=2^0
  Abs : Abs
  Abs1 : Abs
  Add : Sum  Inputs=+-  OutDataType=sfix(16)  OutScaling=2^-10
  Add1 : Sum  Inputs=+-  OutDataType=sfix(16)  OutScaling=2^-10
  Add2 : Sum  OutDataType=sfix(16)  OutScaling=2^-10
  Bus Creator : BusCreator  Inputs=5
  Data Type Conversion{,1..3} (4 alike) : DataTypeConversion  OutDataType=sfix(16)  OutScaling=2^0
  Delay : Constant  Value=0  OutDataType=sfix(16)  OutScaling=2^0
  Divide1 : Product  Inputs=**/  OutDataType=sfix(16)  OutScaling=2^-10
  Max : Constant  Value=100  OutDataType=sfix(16)  OutScaling=2^0
  Relational Operator : RelationalOperator  Operator=<=  LogicOutDataTypeMode=boolean
  Relative Tolerance : Constant  OutDataType=sfix(16)  OutScaling=2^0
  V : Outport  OutDataType=sfix(16)  OutScaling=2^0  InitialOutput=[2]
  wires:
  Abs/1 -> Relational Operator/1
  Add/1 -> Abs/1
  Signal/1 -> Add/1, Data Type Conversion3/1
  Reference/1 -> Add/2, Abs1/1, Add2/2, Add1/1
  Divide1/1 -> Relational Operator/2, Add1/2, Add2/1
  Max/1 -> Divide1/3
  Relative Tolerance/1 -> Divide1/2
  Relational Operator/1 -> Data Type Conversion/1
  Abs1/1 -> Divide1/1
  Delay/1 -> Bus Creator/5  "Delay"
  Add2/1 -> Data Type Conversion2/1
  Add1/1 -> Data Type Conversion1/1
  Bus Creator/1 -> V/1
  Data Type Conversion/1 -> Bus Creator/1  "Local verdict"
  Data Type Conversion1/1 -> Bus Creator/2  "Expected lower limit"
  Data Type Conversion2/1 -> Bus Creator/3  "Expected upper limit"
  Data Type Conversion3/1 -> Bus Creator/4  "Actual data"

== system MIL_Test/Validation Function/Signal comparison/Range - Gap Relative tolerance Precond ==
  Signal : Inport  OutDataType=sfix(16)  OutScaling=2^0
  Reference : Inport  Port=2  OutDataType=sfix(16)  OutScaling=2^0
  Abs : Abs
  Abs1 : Abs
  Add : Sum  Inputs=+-  OutDataType=sfix(16)  OutScaling=2^-10
  Divide1 : Product  Inputs=**/  OutDataType=sfix(16)  OutScaling=2^-10
  Max : Constant  Value=100  OutDataType=sfix(16)  OutScaling=2^0
  Relational Operator : RelationalOperator  Operator=<=  LogicOutDataTypeMode=boolean
  Relative Tolerance : Constant  OutDataType=sfix(16)  OutScaling=2^0
  Activate : Outport  OutDataType=sfix(16)  OutScaling=2^0
  wires:
  Abs1/1 -> Divide1/1
  Relational Operator/1 -> Activate/1
  Relative Tolerance/1 -> Divide1/2
  Max/1 -> Divide1/3
  Divide1/1 -> Relational Operator/2
  Reference/1 -> Abs1/1, Add/2
  Signal/1 -> Add/1
  Add/1 -> Abs/1
  Abs/1 -> Relational Operator/1

== system MIL_Test/Validation Function/Signal comparison/Range - Gap Tolerance range Ass ==
  Signal : Inport  OutDataType=sfix(16)  OutScaling=2^0
  Lower bound : Inport  Port=2  OutDataType=sfix(16)  OutScaling=2^0
  Upper bound : Inport  Port=3  OutDataType=sfix(16)  OutScaling=2^0
  Bus Creator : BusCreator  Inputs=5
  Data Type Conversion{,1..3} (4 alike) : DataTypeConversion  OutDataType=sfix(16)  OutScaling=2^0
  Delay : Constant  Value=0  OutDataType=sfix(16)  OutScaling=2^0
  Logical Operator : Logic  AllPortsSameDT=off  OutDataTypeMode=Specify via dialog
  Relational Operator : RelationalOperator  LogicOutDataTypeMode=boolean
  Relational Operator1 : RelationalOperator  LogicOutDataTypeMode=boolean
  V : Outport  OutDataType=sfix(16)  OutScaling=2^0  InitialOutput=[2]
  wires:
  Upper bound/1 -> Relational Operator1/1, Data Type Conversion2/1
  Relational Operator/1 -> Logical Operator/2
  Relational Operator1/1 -> Logical Operator/1
  Signal/1 -> Relational Operator/1, Relational Operator1/2, Data Type Conversion3/1
  Logical Operator/1 -> Data Type Conversion/1
  Lower bound/1 -> Relational Operator/2, Data Type Conversion1/1
  Delay/1 -> Bus Creator/5  "Delay"
  Bus Creator/1 -> V/1
  Data Type Conversion/1 -> Bus Creator/1  "Local verdict"
  Data Type Conversion1/1 -> Bus Creator/2  "Expected lower limit"
  Data Type Conversion2/1 -> Bus Creator/3  "Expected upper limit"
  Data Type Conversion3/1 -> Bus Creator/4  "Actual data"

== system MIL_Test/Validation Function/Signal comparison/Range - Gap Tolerance range Precond ==
  Signal : Inport  OutDataType=sfix(16)  OutScaling=2^0
  Lower bound : Inport  Port=2  OutDataType=sfix(16)  OutScaling=2^0
  Upper bound : Inport  Port=3  OutDataType=sfix(16)  OutScaling=2^0
  Logical Operator : Logic  AllPortsSameDT=off  OutDataTypeMode=Specify via dialog
  Relational Operator : RelationalOperator  LogicOutDataTypeMode=boolean
  Relational Operator1 : RelationalOperator  LogicOutDataTypeMode=boolean
  Activate : Outport  OutDataType=sfix(16)  OutScaling=2^0
  wires:
  Lower bound/1 -> Relational Operator/2
  Logical Operator/1 -> Activate/1
  Signal/1 -> Relational Operator1/2, Relational Operator/1
  Relational Operator1/1 -> Logical Operator/1
  Relational Operator/1 -> Logical Operator/2
  Upper bound/1 -> Relational Operator1/1

== system MIL_Test/Validation Function/TODO/<system name> ==
  InOut Bus : Inport  OutDataType=sfix(16)  OutScaling=2^0
  <Requirement name> : Subsystem  Description=Requirement template. Create a new requirement from this template.
  Bus Creator : BusCreator  Inputs=1
  Signal Conversion : SignalConversion  ConversionOutput=Bus copy
  Terminator : Terminator
  wires:
  InOut Bus/1 -> Signal Conversion/1
  Bus Creator/1 -> Terminator/1
  <Requirement name>/1(Test Info) -> Bus Creator/1
  Signal Conversion/1 -> <Requirement name>/1(InOut Bus)

== system MIL_Test/Validation Function/TODO/Assertions ==
  Activate : Inport  OutDataType=sfix(16)  OutScaling=2^0
  InOut Bus : Inport  Port=2  OutDataType=sfix(16)  OutScaling=2^0
  Fault info : Subsystem  TreatAsAtomicUnit=on  mask{Ass=[65   99   99   80  101  100   97  108   32   61   61   32   49], Pre=[73  110   79  117  116   10   66  117  115], Req=[83   82   45   80   73   45   48   49   46   51   10   65   99   99  101  108  101  114   97  116  105  111  110   10   80  101  100   97  108   32  114  101   99  111  103  110  105  116  105  111  110]}
      mask prompts: Req "Mask Parameter 3:"
      mask init:
      | set_param(gcb, ...
      |           'Ass', ...
      |           ['[' num2str(uint8(get_param(get_param(gcb,'Parent'),'Name'))) ']']);
      | LinesToAss = getfield(get_param(get_param(get_param(gcb,'Parent'),'handle'),'LineHandles'),'Inport');
      | LinePreToAss = LinesToAss(1);
      | set_param(gcb, ...
      |           'Pre', ...
      |           ['[' num2str(uint8(get_param(get_param(LinePreToAss,'SrcBlockHandle'),'Name'))) ']']); 
      | set_param(gcb, ...
      |           'Req', ...
      |           ['[' num2str(uint8(get_param(get_param(get_param(get_param(gcb,'Parent'),'handle'),'Parent'),'Name'))) ']']);
      | clear LinesToAss LinePreToAss;
  Signal comparison : Subsystem
  VF info : Outport  OutDataType=sfix(16)  OutScaling=2^0

== system MIL_Test/Validation Function/TODO/Model Info ==
  EmptySubsystem : Subsystem

== system MIL_Test/Validation Function/TODO/Preconditions ==
  Signal comparison : Subsystem

== system MIL_Test/Validation Function/TODO/TD determinate (TD D) ==
  Signal : Inport  OutDataType=sfix(16)  OutScaling=2^0
  Trigger : Outport  OutDataType=sfix(16)  OutScaling=2^0
  Feature : Outport  Port=2  OutDataType=sfix(16)  OutScaling=2^0

== system MIL_Test/Validation Function/TODO/TD immediate (TD I) ==
  Signal : Inport  OutDataType=sfix(16)  OutScaling=2^0
  Trigger : Outport  OutDataType=sfix(16)  OutScaling=2^0
  Feature : Outport  Port=2  OutDataType=sfix(16)  OutScaling=2^0

== system MIL_Test/Validation Function/TODO/TD indeterminate ==
  Signal : Inport  OutDataType=sfix(16)  OutScaling=2^0
  R : Outport  OutDataType=sfix(16)  OutScaling=2^0
  T : Outport  Port=2  OutDataType=sfix(16)  OutScaling=2^0
  Feature : Outport  Port=3  OutDataType=sfix(16)  OutScaling=2^0

== system MIL_Test/Validation Function/TODO/TD indeterminate, limited (TD IL) ==
  Signal : Inport  OutDataType=sfix(16)  OutScaling=2^0
  R : Outport  OutDataType=sfix(16)  OutScaling=2^0
  T : Outport  Port=2  OutDataType=sfix(16)  OutScaling=2^0
  Feature : Outport  Port=3  OutDataType=sfix(16)  OutScaling=2^0

== system MIL_Test/Validation Function/TODO/TI determinate (TI D) ==
  Signal : Inport  OutDataType=sfix(16)  OutScaling=2^0
  Feature : Outport  OutDataType=sfix(16)  OutScaling=2^0

== system MIL_Test/Validation Function/TODO/TI immediate (TI I) ==
  Signal : Inport  OutDataType=sfix(16)  OutScaling=2^0
  Feature : Outport  OutDataType=sfix(16)  OutScaling=2^0
